simulink model "ad9361_LTE2"  (R2014b)
settings: Solver=ode45  StartTime=0.0  StopTime=0.1  RelTol=1e-3
PreLoadFcn:
  | load('LTEI.mat');
  | load('LTEQ.mat');
StopFcn:
  | LTEReceiver
libraries: dspsrcs4 x2, simulink x2, simeventslib x1
settings Model: Creator=ACozma  LastModifiedBy=DPu1
settings DebuggingCC: UnderspecifiedInitializationDetection=Classic  MergeDetectMultiDrivingBlocksExec=none

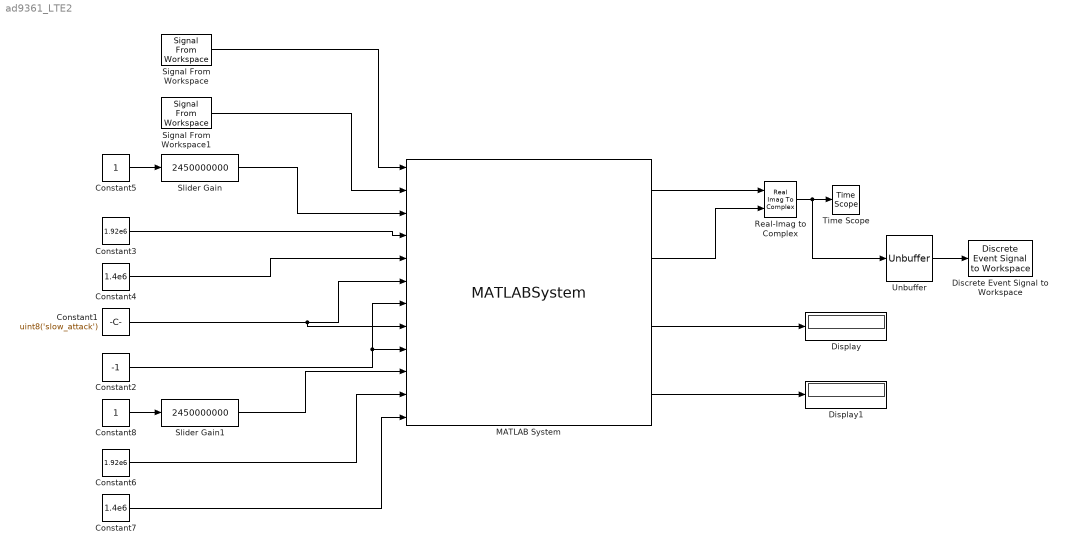
== system ad9361_LTE2 ==
  Constant1 : Constant  Value=uint8('slow_attack')  SampleTime=-1
  Constant2 : Constant  Value=-1  SampleTime=-1
  Constant3 : Constant  Value=1.92e6  SampleTime=-1
  Constant4 : Constant  Value=1.4e6  SampleTime=-1
  Constant5 : Constant  SampleTime=-1
  Constant6 : Constant  Value=1.92e6  SampleTime=-1
  Constant7 : Constant  Value=1.4e6  SampleTime=-1
  Constant8 : Constant  SampleTime=-1
  Discrete Event Signal to Workspace : simeventslib/SimEvents Sinks/Discrete Event Signal to Workspace  VariableName=Rx  SaveFormat=Array  isMonitorOnly=off  isRecordIC=off
      settings: MaxDataPoints=19200*5
  Display : Display
  Display1 : Display
  MATLAB System : MATLABSystem  DialogController=sysobjdialog.BlockDynDialog  System=iio_sys_obj  SimulateUsing=Interpreted execution  ip_address=10.66.99.199  dev_name=ad9361  in_ch_no=2  in_ch_size=19200  out_ch_no=2  out_ch_size=96000
      mask Type: iio_sys_obj
      mask Display:
      | disp('ad9361');
      | port_label('input',1,'DATA_IN1');
      | port_label('input',2,'DATA_IN2');
      | port_label('input',3,'RX_LO_FREQ');
      | port_label('input',4,'RX_SAMPLING_FREQ');
      | port_label('input',5,'RX_RF_BANDWIDTH');
      | port_label('input',6,'RX1_GAIN_MODE');
      | port_label('input',7,'RX1_GAIN');
      | port_label('input',8,'RX2_GAIN_MODE');
      | port_label('input',9,'RX2_GAIN');
      | port_label('input',10,'TX_LO_FREQ');
      | port_label('input',11,'TX_SAMPLING_FREQ');
      | port_label('input',12,'TX_RF_BANDWIDTH');
      | port_label('output',1,'DATA_OUT1');
      | port_label('output',2,'DATA_OUT2');
      | port_label('output',3,'RX1_RSSI');
      | port_label('output',4,'RX2_RSSI');
  Real-Imag to Complex : RealImagToComplex
  Signal From Workspace : dspsrcs4/Signal From Workspace  X=LTEI  Ts=1/1.92e6  nsamps=19200  OutputAfterFinalValue=Cyclic repetition  ignoreOrWarnInputAndFrameLengths=off
  Signal From Workspace1 : dspsrcs4/Signal From Workspace  X=LTEQ  Ts=1/1.92e6  nsamps=19200  OutputAfterFinalValue=Cyclic repetition  ignoreOrWarnInputAndFrameLengths=off
  Slider Gain : simulink/Math Operations/Slider Gain  low=200000  gain=2450000000  high=6000000000
  Slider Gain1 : simulink/Math Operations/Slider Gain  low=200000  gain=2450000000  high=6000000000
  Time Scope : TimeScope  DefaultConfigurationName=spbscopes.TimeScopeBlockCfg
  Unbuffer : Unbuffer  SampleBasedProcessing=Same as frame based
  wires:
  Constant5/1 -> Slider Gain/1
  Constant8/1 -> Slider Gain1/1
  MATLAB System/1 -> Real-Imag to Complex/1
  MATLAB System/2 -> Real-Imag to Complex/2
  Real-Imag to Complex/1 -> Unbuffer/1, Time Scope/1
  MATLAB System/3 -> Display/1
  MATLAB System/4 -> Display1/1
  Slider Gain/1 -> MATLAB System/3
  Constant3/1 -> MATLAB System/4
  Constant4/1 -> MATLAB System/5
  Constant1/1 -> MATLAB System/8, MATLAB System/6
  Constant2/1 -> MATLAB System/9, MATLAB System/7
  Slider Gain1/1 -> MATLAB System/10
  Constant6/1 -> MATLAB System/11
  Constant7/1 -> MATLAB System/12
  Signal From Workspace1/1 -> MATLAB System/2
  Signal From Workspace/1 -> MATLAB System/1
  Unbuffer/1 -> Discrete Event Signal to Workspace/1
